simulink model "tutorial29_control_compare"  (R2025a)
settings: Solver=VariableStepAuto  StartTime=0.0  StopTime=10.0  RelTol=1e-3
libraries: slpidlib x1, simulink x1
settings Model: Creator=xing2  LastModifiedBy=xing2

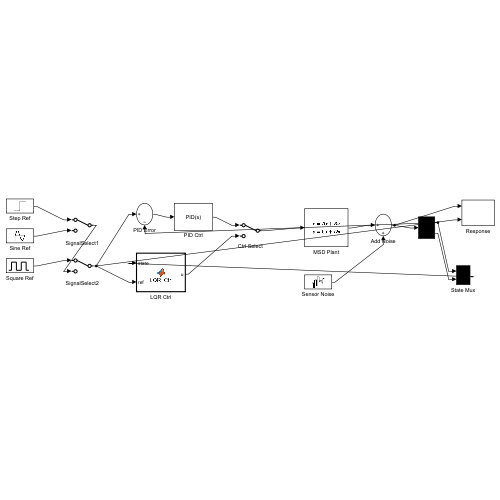
[thumbnail: Simulink's stored preview of the top-level diagram]
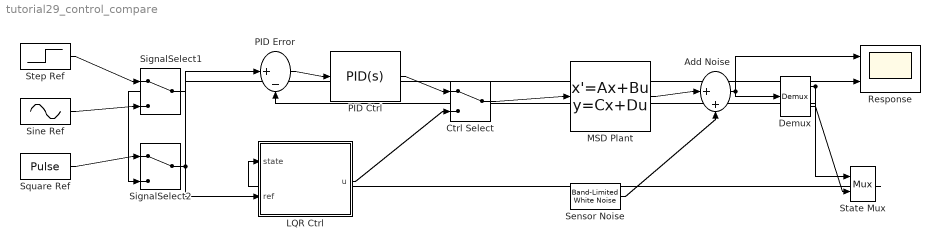
== system tutorial29_control_compare ==
  Add Noise : Sum  Inputs=|++
  Ctrl Select : ManualSwitch
  Demux : Demux  Outputs=2
  LQR Ctrl : MATLAB Function  TreatAsAtomicUnit=on
  MSD Plant : StateSpace  A=[0, 1; -10.0, -0.5]  B=[0; 1]  C=eye(2)  D=[0; 0]  InitialCondition=[0; 0]
  PID Ctrl : slpidlib/PID Controller  Controller=PID  Form=Parallel  TimeDomain=Continuous-time  UseExternalTs=off  SampleTime=-1  IntegratorMethod=Forward Euler  FilterMethod=Forward Euler  ControllerParametersSource=internal  P=50  I=20  UseKiTs=off  D=5  UseExternalDerivativeSource=off  N=100  UseFilter=on  TunerSelectOption=Transfer Function Based (PID Tuner App)  InitialConditionSource=internal  InitialConditionForIntegrator=0  InitialConditionForFilter=0  DifferentiatorICPrevScaledInput=0  ExternalReset=none  TrackingMode=off  Kt=1  LimitOutput=off  SatLimitsSource=internal  UpperSaturationLimit=inf  LowerSaturationLimit=-inf  LinearizeAsGain=on  AntiWindupMode=none  Kb=1  LimitIntegrator=off  UpperIntegratorSaturationLimit=inf  LowerIntegratorSaturationLimit=-inf  POutMin=[]  POutMax=[]  IOutMin=[]  IOutMax=[]  DOutMin=[]  DOutMax=[]  NOutMin=[]  NOutMax=[]  SumOutMin=[]  SumOutMax=[]  SaturationOutMin=[]  SaturationOutMax=[]  PParamMin=[]  PParamMax=[]  IParamMin=[]  IParamMax=[]  DParamMin=[]  DParamMax=[]  NParamMin=[]  NParamMax=[]  KbParamMin=[]  KbParamMax=[]  KtParamMin=[]  KtParamMax=[]  KbOutMin=[]  KbOutMax=[]  KtOutMin=[]  KtOutMax=[]  IntegratorOutMin=[]  IntegratorOutMax=[]  FilterOutMin=[]  FilterOutMax=[]  SumI1OutMin=[]  SumI1OutMax=[]  SumI2OutMin=[]  SumI2OutMax=[]  SumI3OutMin=[]  SumI3OutMax=[]  SumI4OutMin=[]  SumI4OutMax=[]  SumDOutMin=[]  SumDOutMax=[]  DifferentiatorOutMin=[]  DifferentiatorOutMax=[]  FilterDiffOutCoefMin=[]  FilterDiffOutCoefMax=[]  ReciprocalOutMin=[]  ReciprocalOutMax=[]  SumDenOutMin=[]  SumDenOutMax=[]  SumNumOutMin=[]  SumNumOutMax=[]  DivideOutMin=[]  DivideOutMax=[]  UdiffTsProdOutMin=[]  UdiffTsProdOutMax=[]  NTsProdOutMin=[]  NTsProdOutMax=[]  UintegralTsProdOutMin=[]  UintegralTsProdOutMax=[]  UngainTsProdOutMin=[]  UngainTsProdOutMax=[]  ClampingZeroOutDataTypeStr=Inherit: Inherit via back propagation  ClampingZeroOutMin=[]  ClampingZeroOutMax=[]  FilterDenConstantOutDataTypeStr=Inherit: Inherit via back propagation  FilterDenConstantOutMin=[]  FilterDenConstantOutMax=[]  PCopyOutDataTypeStr=Inherit: Inherit via back propagation  PCopyOutMin=[]  PCopyOutMax=[]  NCopyOutDataTypeStr=Inherit: Inherit via back propagation  NCopyOutMin=[]  NCopyOutMax=[]  IntegratorContinuousStateAttributes=''  IntegratorStateMustResolveToSignalObject=off  IntegratorRTWStateStorageClass=Auto  FilterContinuousStateAttributes=''  FilterStateMustResolveToSignalObject=off  FilterRTWStateStorageClass=Auto  ParallelPVariant=InternalParameters  IdealPVariant=Disabled  IVariant=InternalParameters  DVariant=InternalParameters  IntegratorVariant=Continuous  SatVariant=Disabled  AWVariant=Passthrough  PCopyVariant=Disabled  TRVariant=Disabled  FdbkBlocksVariant=Forward  IdealPFdbkVariant=Disabled  SatFdbkVariant=Disabled  DerivativeFilterVariant=ContFilter  NVariant=InternalParameters  NCopyVariant=Disabled  FilterICVariant=InternalICsFilter  IntegratorICVariant=InternalICs  ExternalResetVariant=Disabled  TRSumVariant=Passthrough  SumFdbkVariant=Disabled  SumVariant=Sum_PID  TsampFilterVariant=InternalTs  TsampNgainVariant=Passthrough  TsampIntegralVariant=Disabled_SignalSpec  ExternalSaturationOutDataTypeStr=Inherit: Same as second input  DerivativeSourceVariant=ErrorSignal  PreIntVariant=InternalPreInt
  PID Error : Sum  Inputs=|+-
  Response : Scope  NumInputPorts=2
  Sensor Noise : simulink/Sources/Band-Limited White Noise  Cov=[0.1]  Ts=0.1  seed=[23341]
  SignalSelect1 : ManualSwitch
  SignalSelect2 : ManualSwitch
  Sine Ref : Sin  Amplitude=0.5  Frequency=5  SampleTime=0
  Square Ref : DiscretePulseGenerator  PulseType=Time based  PulseWidth=5
  State Mux : Mux  Inputs=2
  Step Ref : Step  Time=0.2  SampleTime=0
  wires:
  Step Ref/1 -> SignalSelect1/1
  Sine Ref/1 -> SignalSelect1/2
  SignalSelect1/1 -> SignalSelect2/2
  Square Ref/1 -> SignalSelect2/1
  SignalSelect2/1 -> PID Error/1, LQR Ctrl/2(ref), Response/2
  PID Error/1 -> PID Ctrl/1
  PID Ctrl/1 -> Ctrl Select/1
  LQR Ctrl/1(u) -> Ctrl Select/2
  Ctrl Select/1 -> MSD Plant/1
  MSD Plant/1 -> Add Noise/1
  Sensor Noise/1 -> Add Noise/2
  Add Noise/1 -> Demux/1, Response/1
  Demux/1 -> PID Error/2, State Mux/1
  Demux/2 -> State Mux/2
  State Mux/1 -> LQR Ctrl/1(state)

== matlab function tutorial29_control_compare/LQR Ctrl ==
  data: state input; u output; ref input
function u = LQR_Ctrl(state, ref)
% LQR 最优控制律: u = -K1*(x1-ref) - K2*x2
K = [23.17, 7.02];
u = -K(1)*(state(1)-ref) - K(2)*state(2);
u = max(min(u, 10), -10);   % 限幅
